simulink model "tether000_th"  (R2018b)
settings: Solver=VariableStepAuto  StartTime=0.0  StopTime=10.0  RelTol=1e-3
libraries: tethers_cl x1
settings Model: Creator=mcobb  LastModifiedBy=mcobb

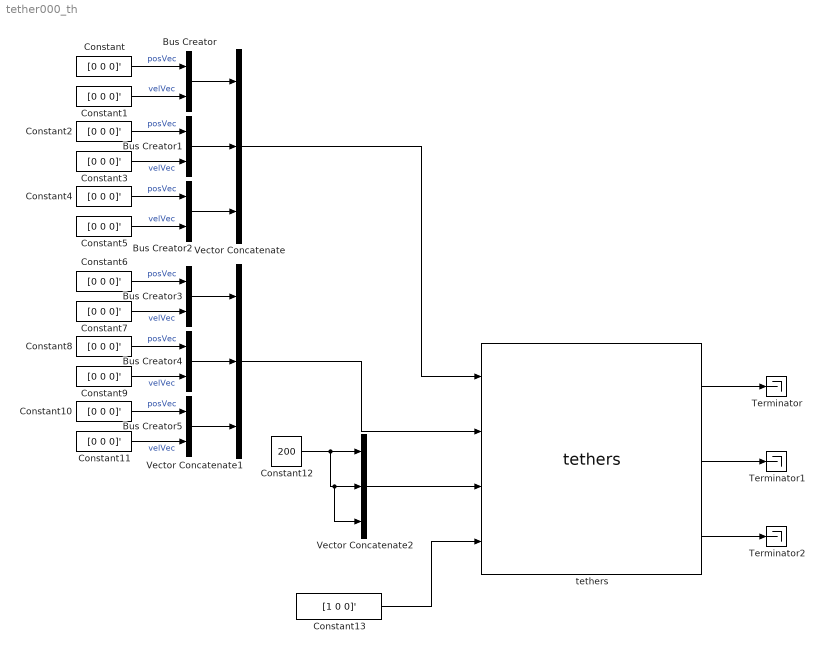
== system tether000_th ==
  Bus Creator{,1..5} (6 alike) : BusCreator  Inputs=2
  Constant{,1..11} (12 alike) : Constant  Value=[0 0 0]'
  Constant12 : Constant  Value=200
  Constant13 : Constant  Value=[1 0 0]'
  Terminator : Terminator
  Terminator1 : Terminator
  Terminator2 : Terminator
  Vector Concatenate : Concatenate  NumInputs=3
  Vector Concatenate1 : Concatenate  NumInputs=3
  Vector Concatenate2 : Concatenate  NumInputs=3
  tethers : tethers_cl/tethers  thr=thr
  wires:
  Constant/1 -> Bus Creator/1  "posVec"
  Constant1/1 -> Bus Creator/2  "velVec"
  Constant3/1 -> Bus Creator1/2  "velVec"
  Constant2/1 -> Bus Creator1/1  "posVec"
  Constant4/1 -> Bus Creator2/1  "posVec"
  Constant5/1 -> Bus Creator2/2  "velVec"
  Constant11/1 -> Bus Creator5/2  "velVec"
  Constant10/1 -> Bus Creator5/1  "posVec"
  Constant8/1 -> Bus Creator4/1  "posVec"
  Constant9/1 -> Bus Creator4/2  "velVec"
  Constant7/1 -> Bus Creator3/2  "velVec"
  Constant6/1 -> Bus Creator3/1  "posVec"
  Bus Creator1/1 -> Vector Concatenate/2
  Bus Creator/1 -> Vector Concatenate/1
  Bus Creator2/1 -> Vector Concatenate/3
  Bus Creator4/1 -> Vector Concatenate1/2
  Bus Creator3/1 -> Vector Concatenate1/1
  Bus Creator5/1 -> Vector Concatenate1/3
  Vector Concatenate/1 -> tethers/1
  Vector Concatenate1/1 -> tethers/2
  Vector Concatenate2/1 -> tethers/3
  Constant12/1 -> Vector Concatenate2/3, Vector Concatenate2/2, Vector Concatenate2/1
  Constant13/1 -> tethers/4
  tethers/1 -> Terminator/1
  tethers/3 -> Terminator2/1
  tethers/2 -> Terminator1/1
